simulink model "ConvertidorBUCKBIDIRECCIONAL_Arreglado"  (R2024b)
settings: Solver=VariableStepAuto  StartTime=0.0  StopTime=.5  RelTol=1e-3
libraries: spsSeriesRLCBranchLib x5, spsMultimeterLib x5, spsIdealSwitchLib x4, spsDCVoltageSourceLib x2, spsMosfetLib x2, sps_lib x1
settings Model: Creator=ignac  LastModifiedBy=ignac

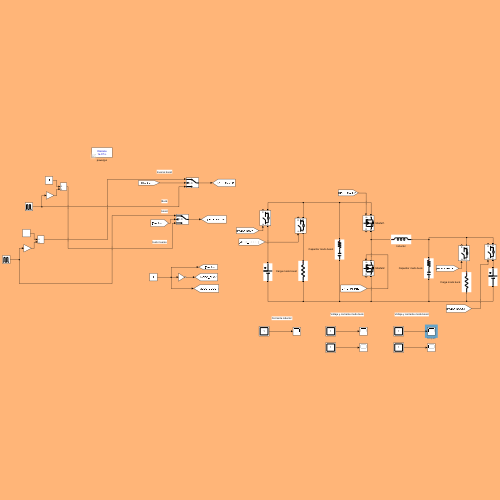
[thumbnail: Simulink's stored preview of the top-level diagram]
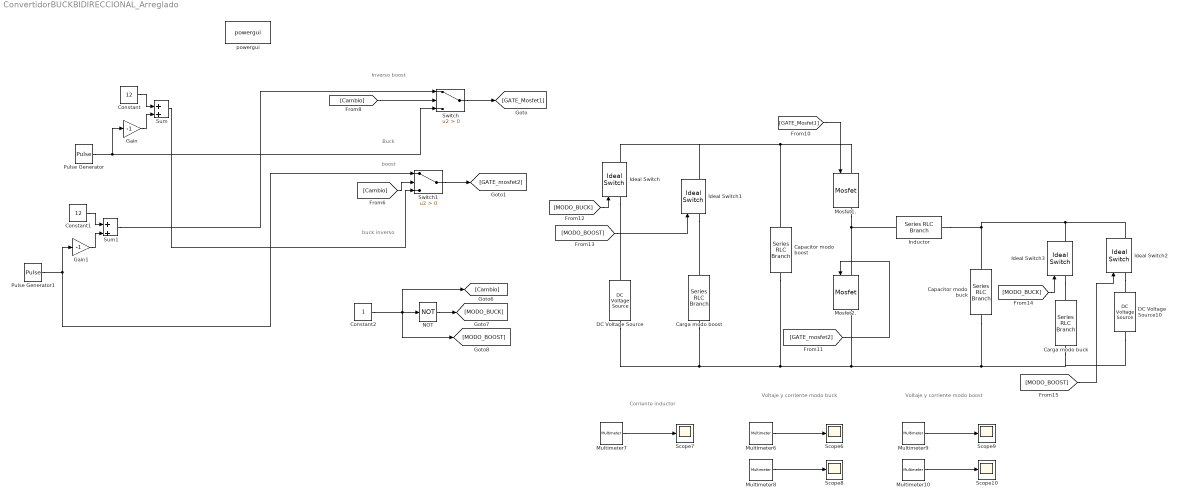
== system ConvertidorBUCKBIDIRECCIONAL_Arreglado ==
  note: buck inverso
  note: boost
  note: Inverso boost
  note: Buck
  note: Corriente inductor
  note: Voltaje y corriente modo buck
  note: Voltaje y corriente modo boost
  Capacitor modo boost : spsSeriesRLCBranchLib/Series RLC Branch  LConnTagsString=__new0  RConnTagsString=__new0  BranchType=RC  Resistance=1  Inductance=1e-3  SetiL0=off  InitialCurrent=0  Capacitance=6.35e-6  Setx0=off  InitialVoltage=0  Measurements=None
  Capacitor modo buck : spsSeriesRLCBranchLib/Series RLC Branch  LConnTagsString=__new0  RConnTagsString=__new0  BranchType=RC  Resistance=1  Inductance=1e-3  SetiL0=off  InitialCurrent=0  Capacitance=1.6e-6  Setx0=off  InitialVoltage=0  Measurements=Branch voltage
  Carga modo boost : spsSeriesRLCBranchLib/Series RLC Branch  LConnTagsString=__new0  RConnTagsString=__new0  BranchType=R  Resistance=145.8  Inductance=1e-3  SetiL0=off  InitialCurrent=0  Capacitance=1e-6  Setx0=off  InitialVoltage=0  Measurements=Branch voltage and current
  Carga modo buck : spsSeriesRLCBranchLib/Series RLC Branch  LConnTagsString=__new0  RConnTagsString=__new0  BranchType=R  Resistance=39.2  Inductance=1e-3  SetiL0=off  InitialCurrent=0  Capacitance=1e-6  Setx0=off  InitialVoltage=0  Measurements=Branch voltage and current
  Constant : Constant  Value=12
  Constant1 : Constant  Value=12
  Constant2 : Constant
  DC Voltage Source : spsDCVoltageSourceLib/DC Voltage Source  Amplitude=23  Measurements=None
  DC Voltage Source10 : spsDCVoltageSourceLib/DC Voltage Source  Amplitude=12  Measurements=None
  Gain : Gain  Gain=-1
  Gain1 : Gain  Gain=-1
  Ideal Switch{,1..3} (4 alike) : spsIdealSwitchLib/Ideal Switch  Ron=0.001  Lon=0  IC=0  Rs=1e5  Cs=inf  Measurements=on
  Inductor : spsSeriesRLCBranchLib/Series RLC Branch  LConnTagsString=__new0  RConnTagsString=__new0  BranchType=L  Resistance=1  Inductance=1e-3  SetiL0=off  InitialCurrent=0  Capacitance=1e-6  Setx0=off  InitialVoltage=0  Measurements=Branch current
  Mosfet1. : spsMosfetLib/Mosfet  Ron=22e-3  Lon=0  Rd=0.01  Vfd=0  IC=0  Rs=1e5  Cs=inf  Measurements=on
  Mosfet2. : spsMosfetLib/Mosfet  Ron=22e-3  Lon=0  Rd=0.01  Vfd=0  IC=0  Rs=1e5  Cs=inf  Measurements=on
  Multimeter10 : spsMultimeterLib/Multimeter  L=6  sel=4  yselected={}  Gain=1  OutputType=Complex  PlotAtSimulationStop=off  PhasorSimulation=off
  Multimeter6 : spsMultimeterLib/Multimeter  L=6  sel=3  yselected={}  Gain=1  OutputType=Complex  PlotAtSimulationStop=off  PhasorSimulation=off
  Multimeter7 : spsMultimeterLib/Multimeter  L=6  sel=6  yselected={}  Gain=1  OutputType=Complex  PlotAtSimulationStop=off  PhasorSimulation=off
  Multimeter8 : spsMultimeterLib/Multimeter  L=6  sel=5  yselected={}  Gain=1  OutputType=Complex  PlotAtSimulationStop=off  PhasorSimulation=off
  Multimeter9 : spsMultimeterLib/Multimeter  L=6  sel=2  yselected={}  Gain=1  OutputType=Complex  PlotAtSimulationStop=off  PhasorSimulation=off
  NOT : Logic  Operator=NOT  IconShape=distinctive  AllPortsSameDT=off  OutDataTypeStr=boolean
  Pulse Generator : DiscretePulseGenerator  PulseType=Time based  Amplitude=12  Period=1/60000  PulseWidth=60.8
  Pulse Generator1 : DiscretePulseGenerator  PulseType=Time based  Amplitude=12  Period=1/60000  PulseWidth=55.6
  Scope{6..10} (5 alike) : Scope
  Sum : Sum  Inputs=|++
  Sum1 : Sum  Inputs=|++
  Switch : Switch  Criteria=u2 > Threshold  SaturateOnIntegerOverflow=off  InputSameDT=off
  Switch1 : Switch  Criteria=u2 > Threshold  SaturateOnIntegerOverflow=off  InputSameDT=off
  powergui : sps_lib/powergui  Priority=1  SimulationMode=Discrete  SampleTime=1e-7  frequency=60  Iterations=50  frequencyindice=0  Pbase=100e6  ErrMax=1e-4  UnitsV=kV  UnitsW=MW  buscounter=0  FunctionMessages=off  echomessages=off  EnableUseOfTLC=off  CurrentSourceSwitches=off  DisableSnubberDevices=off  DisableRonSwitches=off  DisableVfSwitches=off  DisplayEquations=off  AutomaticDiscreteSolvers=off  SolverType=Tustin/Backward Euler (TBE)  Interpol=off  ExternalGateDelay=off  methode=off  Ts=100  x0status=blocks  SPID=on  SwTol=0  HookPort=off  NonlinearTolerance=1e-4  nMaxIteration=100  ContinueOnMaxIteration=off  RestoreLinks=warning  ResistiveCurrentMeasurement=off  Frange=[0:2:500]  Ylog=off  Xlog=on  ShowGrid=off  save=off  variable=ZData  structure=0  ZoomFFT=off  StartTime=0.0  cycles=1  DisplayStyle=1  fundamental=60  FreqAxis=off  MaxFrequency=1000  frequencyindicesteady=1  RmsSteady=1  display=off
  wires:
  Gain/1 -> Sum/2
  Constant/1 -> Sum/1
  Gain1/1 -> Sum1/2
  Constant1/1 -> Sum1/1
  [Cambio] -> Switch1/2
  Pulse Generator1/1 -> Gain1/1, Switch1/1
  Sum/1 -> Switch1/3
  Switch/1 -> [GATE_Mosfet1]
  Switch1/1 -> [GATE_mosfet2]
  Constant2/1 -> [Cambio], NOT/1, [MODO_BOOST]
  [Cambio] -> Switch/2
  [GATE_Mosfet1] -> Mosfet1./1
  [GATE_mosfet2] -> Mosfet2./1
  [MODO_BUCK] -> Ideal Switch/1
  [MODO_BOOST] -> Ideal Switch1/1
  [MODO_BUCK] -> Ideal Switch3/1
  [MODO_BOOST] -> Ideal Switch2/1
  Multimeter6/1 -> Scope6/1
  Multimeter7/1 -> Scope7/1
  Multimeter8/1 -> Scope8/1
  Multimeter9/1 -> Scope9/1
  Multimeter10/1 -> Scope10/1
  Sum1/1 -> Switch/1
  Pulse Generator/1 -> Switch/3, Gain/1
  NOT/1 -> [MODO_BUCK]
  connections:
  Mosfet1./RConn1 -- Inductor/LConn1 -- Mosfet2./LConn1
  DC Voltage Source/LConn1 -- Mosfet2./RConn1 -- DC Voltage Source10/LConn1 -- Carga modo buck/RConn1 -- Capacitor modo buck/RConn1 -- Capacitor modo boost/RConn1 -- Carga modo boost/RConn1
  Capacitor modo boost/LConn1 -- Ideal Switch1/RConn1 -- Ideal Switch/RConn1 -- Mosfet1./LConn1
  Capacitor modo buck/LConn1 -- Inductor/RConn1 -- Ideal Switch2/RConn1 -- Ideal Switch3/RConn1
  Ideal Switch1/LConn1 -- Carga modo boost/LConn1
  Ideal Switch/LConn1 -- DC Voltage Source/RConn1
  Ideal Switch3/LConn1 -- Carga modo buck/LConn1
  Ideal Switch2/LConn1 -- DC Voltage Source10/RConn1
